simulink model "simul1"  (R2023b)
settings: Solver=ode4  StartTime=0.0  StopTime=600  FixedStep=1/5000  RelTol=1e-3
InitFcn:
  | init1
StopFcn:
  | stop1
values from neighbouring files (symbols this model uses):
  fs = 5000    [init1.m]
settings Model: Creator=xavie  LastModifiedBy=xavie
settings DataIOCC: ReturnWorkspaceOutputs=off

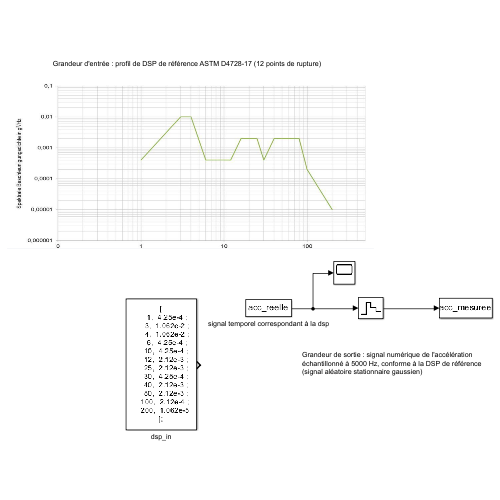
[thumbnail: Simulink's stored preview of the top-level diagram]
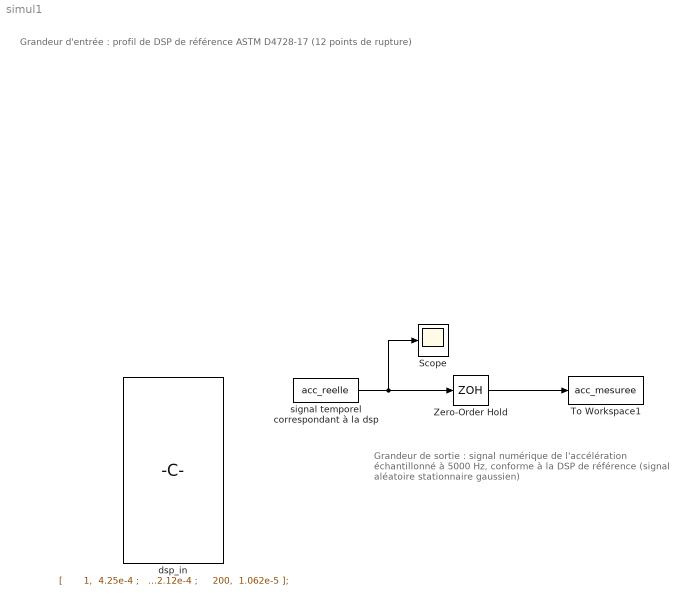
== system simul1 ==
  note: Grandeur de sortie : signal numérique de l'accélération échantillonné à 5000 Hz, conforme à la DSP de référence (signal aléatoire stationnaire gaussien)
  note: Grandeur d'entrée : profil de DSP de référence ASTM D4728-17 (12 points de rupture)
  Scope : Scope
  To Workspace1 : ToWorkspace  VariableName=acc_mesuree  SampleTime=-1
      settings: Save2DSignal=2-D array (concatenate along first dimension)
  Zero-Order Hold : ZeroOrderHold  SampleTime=1/fs
  dsp_in : Constant  Value=|
      | [
      |       1,  4.25e-4 ;
      |       3,  1.062e-2 ;
      |       4,  1.062e-2 ;
      |       6,  4.25e-4 ;
      |      10,  4.25e-4 ;
      |      12,  2.12e-3 ;
      |      25,  2.12e-3 ;
      |      30,  4.25e-4 ;
      |      40,  2.12e-3 ;
      |      80,  2.12e-3 ;
      |     100,  2.12e-4 ;
      |     200,  1.062e-5
      | ];
  signal temporel correspondant à la dsp : FromWorkspace  VariableName=acc_reelle
  wires:
  signal temporel correspondant à la dsp/1 -> Zero-Order Hold/1, Scope/1
  Zero-Order Hold/1 -> To Workspace1/1
